simulink model "Simulink_ejercicio_4"  (R2016b)
settings: Solver=VariableStepAuto  StartTime=0.0  StopTime=200  RelTol=1e-3
values from neighbouring files (symbols this model uses):
  A = [-0.13150 0.14858 0.0 0.32434 -0.93964 ... (first row only)    [ejercicio4.m]
  B = [ 0.00012049 0.00032897 ... (first row only)    [ejercicio4.m]
  C = [0.0 0.0 0.0 180/pi 0.0 ... (first row only)    [ejercicio4.m]
  D = zeros(2,2)    [ejercicio4.m]
  Kp = -0.4    [ejercicio4.m]
  Kr = -1.3    [ejercicio4.m]
  tau_a = 1/20.2    (= 0.049504950495)    [ejercicio4.m]
  tau_r = 1/20.2    (= 0.049504950495)    [ejercicio4.m]
  tau_W = 1    [ejercicio4.m]
settings Model: Creator=inmaculadacoronaperez  LastModifiedBy=Alvaro

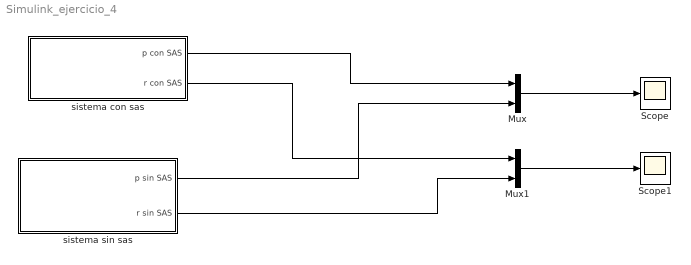
== system Simulink_ejercicio_4 ==
  Mux : Mux  Inputs=2
  Mux1 : Mux  Inputs=2
  Scope : Scope
  Scope1 : Scope
  sistema con sas : Subsystem
  sistema sin sas : Subsystem
  wires:
  sistema con sas/1(p con SAS) -> Mux/1
  sistema sin sas/1(p sin SAS) -> Mux/2
  sistema con sas/2(r con SAS) -> Mux1/1
  sistema sin sas/2(r sin SAS) -> Mux1/2
  Mux1/1 -> Scope1/1
  Mux/1 -> Scope/1

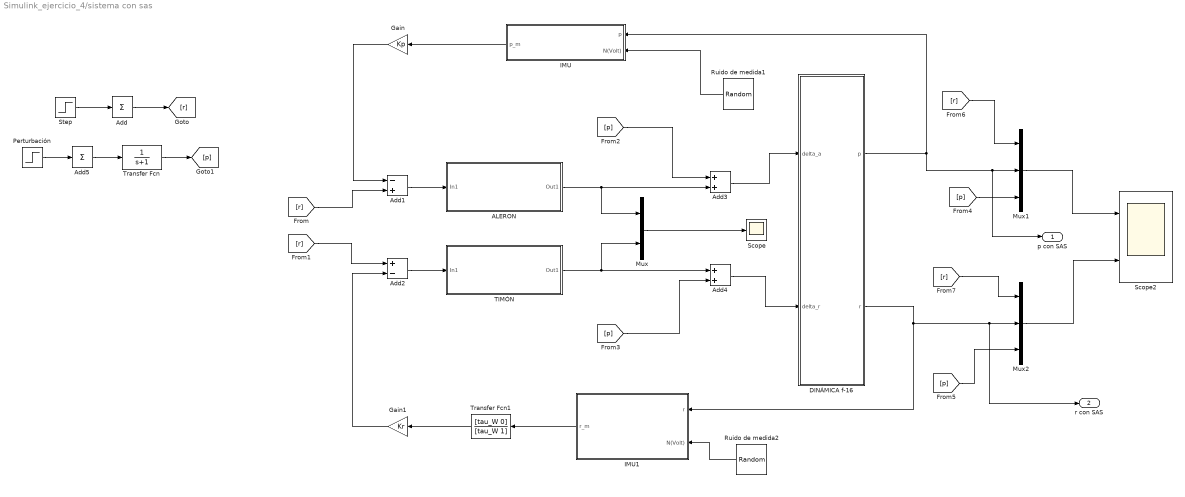
== system Simulink_ejercicio_4/sistema con sas ==
  ALERON : Subsystem
  Add : Sum  Inputs=+
  Add1 : Sum  Inputs=-+
  Add2 : Sum  Inputs=+-
  Add3 : Sum
  Add4 : Sum
  Add5 : Sum  Inputs=+
  DINÁMICA f-16 : Subsystem  mask(Dinámica F-16){A=A, B=B, C=C, D=D, Ci=[0 0 0 0]}
      mask prompts: A "Matriz de estados (A)"; B "Matriz de estados (B)"; C "Matriz de estados (C)"; D "Matriz de estados (D)"; Ci "Condiciones iniciales (nominales)"
  Gain : Gain  Gain=Kp
  Gain1 : Gain  Gain=Kr
  IMU : Subsystem
  IMU1 : Subsystem
  Mux : Mux  Inputs=2
  Mux1 : Mux  Inputs=3
  Mux2 : Mux  Inputs=3
  Perturbación : Step  Time=[30 31 ]  Before=[0 0 ]  After=[0.5 -0.5]  SampleTime=0
  Ruido de medida1 : RandomNumber  Variance=1e-4  Seed=123456  SampleTime=0.01
  Ruido de medida2 : RandomNumber  Variance=1e-5  Seed=123456  SampleTime=0.01
  Scope : Scope
  Scope2 : Scope  NumInputPorts=2
  Step : Step  Time=[10 11]  Before=[0 0]  After=[1 -1]  SampleTime=0
  TIMÓN : Subsystem
  Transfer Fcn : TransferFcn  Denominator=[1 1]
  Transfer Fcn1 : TransferFcn  Numerator=[tau_W 0]  Denominator=[tau_W 1]
  p con SAS : Outport
  r con SAS : Outport  Port=2
  wires:
  TIMÓN/1(Out1) -> Add4/1, Mux/2
  Mux/1 -> Scope/1
  ALERON/1(Out1) -> Add3/2, Mux/1
  Transfer Fcn/1 -> [p]
  [r] -> Add1/2
  [r] -> Add2/1
  Gain/1 -> Add1/1
  Mux2/1 -> Scope2/2
  [p] -> Mux2/3
  [r] -> Mux2/1
  DINÁMICA f-16/1(p) -> p con SAS/1, Mux1/2, IMU/1(p)
  Ruido de medida1/1 -> IMU/2(N(Volt))
  Ruido de medida2/1 -> IMU1/2(N(Volt))
  [p] -> Mux1/3
  DINÁMICA f-16/2(r) -> IMU1/1(r), r con SAS/1, Mux2/2
  Perturbación/1 -> Add5/1
  Add5/1 -> Transfer Fcn/1
  Step/1 -> Add/1
  Add/1 -> [r]
  Mux1/1 -> Scope2/1
  [r] -> Mux1/1
  [p] -> Add3/1
  [p] -> Add4/2
  Gain1/1 -> Add2/2
  Transfer Fcn1/1 -> Gain1/1
  IMU1/1("r_m ") -> Transfer Fcn1/1
  Add2/1 -> TIMÓN/1(In1)
  Add1/1 -> ALERON/1(In1)
  IMU/1("p_m ") -> Gain/1
  Add3/1 -> DINÁMICA f-16/1(delta_a)
  Add4/1 -> DINÁMICA f-16/2(delta_r)

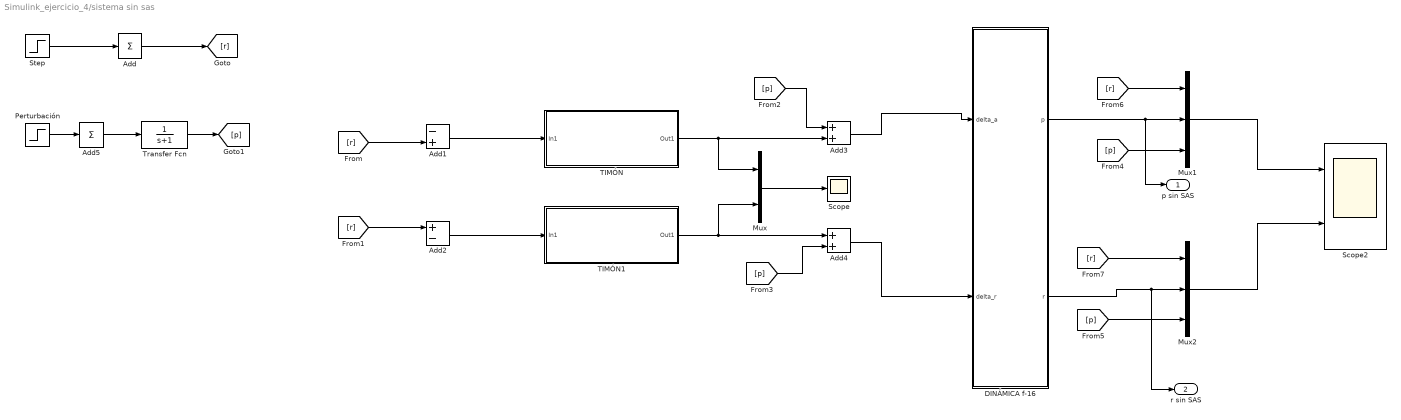
== system Simulink_ejercicio_4/sistema sin sas ==
  Add : Sum  Inputs=+
  Add1 : Sum  Inputs=-+
  Add2 : Sum  Inputs=+-
  Add3 : Sum
  Add4 : Sum
  Add5 : Sum  Inputs=+
  DINÁMICA f-16 : Subsystem  mask(Dinámica F-16){A=A, B=B, C=C, D=D, Ci=[0 0 0 0]}
      mask prompts: A "Matriz de estados (A)"; B "Matriz de estados (B)"; C "Matriz de estados (C)"; D "Matriz de estados (D)"; Ci "Condiciones iniciales (nominales)"
  Mux : Mux  Inputs=2
  Mux1 : Mux  Inputs=3
  Mux2 : Mux  Inputs=3
  Perturbación : Step  Time=[30 31 ]  Before=[0 0 ]  After=[0.5 -0.5]  SampleTime=0
  Scope : Scope
  Scope2 : Scope  NumInputPorts=2
  Step : Step  Time=[10 11]  Before=[0 0]  After=[1 -1]  SampleTime=0
  TIMÓN : Subsystem
  TIMÓN1 : Subsystem
  Transfer Fcn : TransferFcn  Denominator=[1 1]
  p sin SAS : Outport
  r sin SAS : Outport  Port=2
  wires:
  TIMÓN1/1(Out1) -> Add4/1, Mux/2
  Mux/1 -> Scope/1
  Add2/1 -> TIMÓN1/1(In1)
  TIMÓN/1(Out1) -> Add3/2, Mux/1
  Transfer Fcn/1 -> [p]
  [r] -> Add1/2
  [r] -> Add2/1
  Mux2/1 -> Scope2/2
  [p] -> Mux2/3
  [r] -> Mux2/1
  DINÁMICA f-16/1(p) -> p sin SAS/1, Mux1/2
  Add1/1 -> TIMÓN/1(In1)
  [p] -> Mux1/3
  DINÁMICA f-16/2(r) -> r sin SAS/1, Mux2/2
  Perturbación/1 -> Add5/1
  Add5/1 -> Transfer Fcn/1
  Step/1 -> Add/1
  Add/1 -> [r]
  Mux1/1 -> Scope2/1
  [r] -> Mux1/1
  [p] -> Add3/1
  [p] -> Add4/2
  Add3/1 -> DINÁMICA f-16/1(delta_a)
  Add4/1 -> DINÁMICA f-16/2(delta_r)

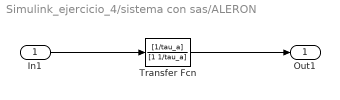
== system Simulink_ejercicio_4/sistema con sas/ALERON ==
  In1 : Inport
  Transfer Fcn : TransferFcn  Numerator=[1/tau_a]  Denominator=[1 1/tau_a]
  Out1 : Outport
  wires:
  In1/1 -> Transfer Fcn/1
  Transfer Fcn/1 -> Out1/1

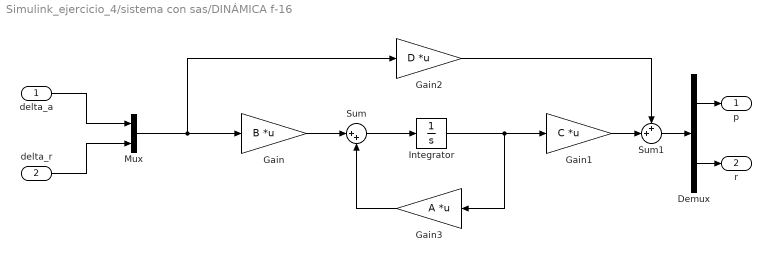
== system Simulink_ejercicio_4/sistema con sas/DINÁMICA f-16 ==
  delta_a : Inport
  delta_r : Inport  Port=2
  Demux : Demux  Outputs=2
  Gain : Gain  Gain=B  Multiplication=Matrix(K*u)
  Gain1 : Gain  Gain=C  Multiplication=Matrix(K*u)
  Gain2 : Gain  Gain=D  Multiplication=Matrix(K*u)
  Gain3 : Gain  Gain=A  Multiplication=Matrix(K*u)
  Integrator : Integrator
  Mux : Mux  Inputs=2
  Sum : Sum  Inputs=|++
  Sum1 : Sum  Inputs=++|
  p : Outport
  r : Outport  Port=2
  wires:
  Gain/1 -> Sum/1
  Sum/1 -> Integrator/1
  Integrator/1 -> Gain3/1, Gain1/1
  Gain2/1 -> Sum1/1
  Gain3/1 -> Sum/2
  Gain1/1 -> Sum1/2
  Demux/1 -> p/1
  Demux/2 -> r/1
  Sum1/1 -> Demux/1
  delta_r/1 -> Mux/2
  delta_a/1 -> Mux/1
  Mux/1 -> Gain/1, Gain2/1

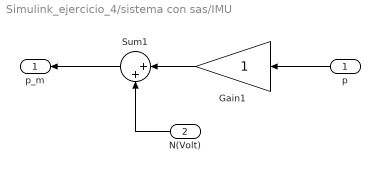
== system Simulink_ejercicio_4/sistema con sas/IMU ==
  p : Inport
  N(Volt) : Inport  Port=2
  Gain1 : Gain
  Sum1 : Sum  Inputs=|++
  "p_m " : Outport
  wires:
  p/1 -> Gain1/1
  Gain1/1 -> Sum1/1
  N(Volt)/1 -> Sum1/2
  Sum1/1 -> "p_m "/1

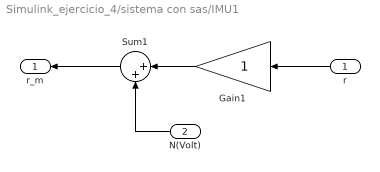
== system Simulink_ejercicio_4/sistema con sas/IMU1 ==
  r : Inport
  N(Volt) : Inport  Port=2
  Gain1 : Gain
  Sum1 : Sum  Inputs=|++
  "r_m " : Outport
  wires:
  r/1 -> Gain1/1
  Gain1/1 -> Sum1/1
  N(Volt)/1 -> Sum1/2
  Sum1/1 -> "r_m "/1

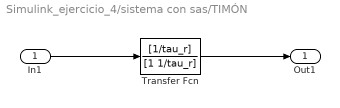
== system Simulink_ejercicio_4/sistema con sas/TIMÓN ==
  In1 : Inport
  Transfer Fcn : TransferFcn  Numerator=[1/tau_r]  Denominator=[1 1/tau_r]
  Out1 : Outport
  wires:
  In1/1 -> Transfer Fcn/1
  Transfer Fcn/1 -> Out1/1

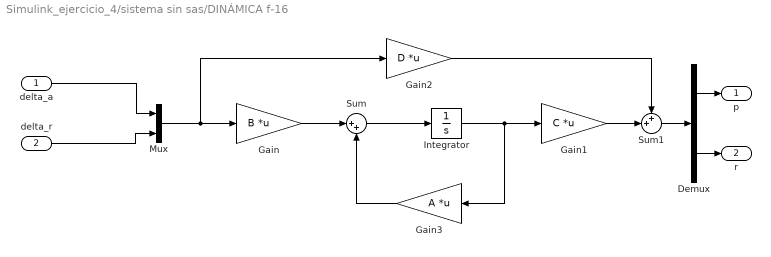
== system Simulink_ejercicio_4/sistema sin sas/DINÁMICA f-16 ==
  delta_a : Inport
  delta_r : Inport  Port=2
  Demux : Demux  Outputs=2
  Gain : Gain  Gain=B  Multiplication=Matrix(K*u)
  Gain1 : Gain  Gain=C  Multiplication=Matrix(K*u)
  Gain2 : Gain  Gain=D  Multiplication=Matrix(K*u)
  Gain3 : Gain  Gain=A  Multiplication=Matrix(K*u)
  Integrator : Integrator
  Mux : Mux  Inputs=2
  Sum : Sum  Inputs=|++
  Sum1 : Sum  Inputs=++|
  p : Outport
  r : Outport  Port=2
  wires:
  Gain/1 -> Sum/1
  Sum/1 -> Integrator/1
  Integrator/1 -> Gain3/1, Gain1/1
  Gain2/1 -> Sum1/1
  Gain3/1 -> Sum/2
  Gain1/1 -> Sum1/2
  Demux/1 -> p/1
  Demux/2 -> r/1
  Sum1/1 -> Demux/1
  delta_r/1 -> Mux/2
  delta_a/1 -> Mux/1
  Mux/1 -> Gain2/1, Gain/1

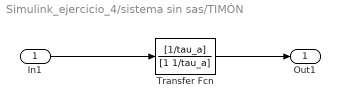
== system Simulink_ejercicio_4/sistema sin sas/TIMÓN ==
  In1 : Inport
  Transfer Fcn : TransferFcn  Numerator=[1/tau_a]  Denominator=[1 1/tau_a]
  Out1 : Outport
  wires:
  In1/1 -> Transfer Fcn/1
  Transfer Fcn/1 -> Out1/1

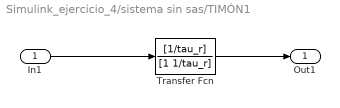
== system Simulink_ejercicio_4/sistema sin sas/TIMÓN1 ==
  In1 : Inport
  Transfer Fcn : TransferFcn  Numerator=[1/tau_r]  Denominator=[1 1/tau_r]
  Out1 : Outport
  wires:
  In1/1 -> Transfer Fcn/1
  Transfer Fcn/1 -> Out1/1
